simulink model "estimator"  (R2024a)
settings: Solver=FixedStepAuto  StartTime=0.0  StopTime=400  FixedStep=0.001  RelTol=1e-3
InitFcn:
  | Kx = 20;
  | Kf = 21;
settings Model: Creator=bemran  LastModifiedBy=bemran

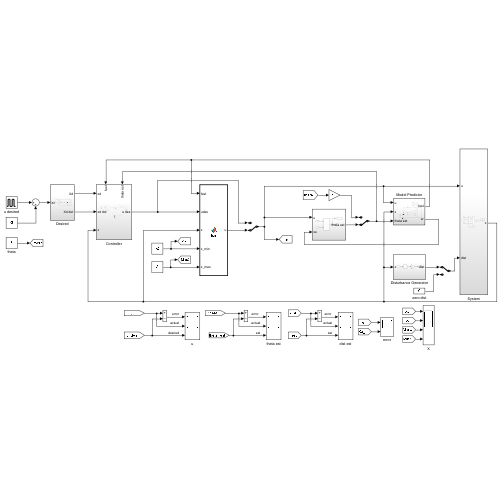
[thumbnail: Simulink's stored preview of the top-level diagram]
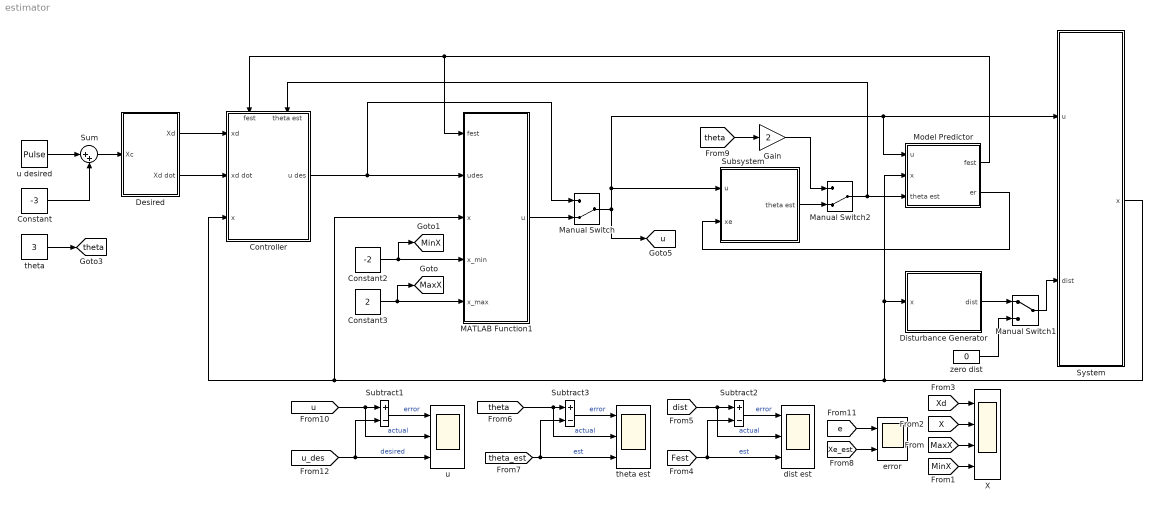
== system estimator ==
  Constant : Constant  Value=-3
  Constant2 : Constant  Value=-2
  Constant3 : Constant  Value=2
  Controller : Subsystem
      settings: PortSchema="{\"entries\":[{\"content\":{\"sides\":[{\"content\":{\"connectorIds\":[\"In1\",\"In2\",\"In3\"]},\"type\":\"ConnectorPlacement.EquallySpacedRectSide\",\"uuid\":\"b6f38cdc-8bf3-4480-b58d-f3be2425ec5d\"},{\"content\":{\"connectorIds\":[\"Out1\"],\"side\":\"RIGHT\"},\"type\":\"ConnectorPlacement.EquallySpacedRectSide\",\"uuid\":\"bcaedb91-bba6-4987-806b-aba45422edc9\"},{\"content\":{\"connectorIds\":[\"In4\",\"In5\"],\"side\":\"TOP\"},\"type\":\"ConnectorPlacement.EquallySpacedRectSide\",\"uuid\":\"b280daf0-8ac8-4898-b226-e1ec0883028d\"},{\"content\":{\"side\":\"BOTTOM\"},\"type\":\"ConnectorPlacement.EquallySpacedRectSide\",\"uuid\":\"a3314033-a6b2-4450-a5a3-9d51c6c5191b\"}]},\"type\":\"ConnectorPlacement.EquallySpacedConnector\",\"uuid\":\"d4e8f3f5-abab-496a-b317-e8d184215eb1\"}],\"packageUris\":[\"http://schema.mathworks.com/mf0/Connector/R2020b\"],\"version\":\"1.0\"}"
  Desired : Subsystem
  Disturbance Generator : Subsystem
  Gain : Gain  Gain=2
  MATLAB Function1 : MATLAB Function  TreatAsAtomicUnit=on
  Manual Switch : ManualSwitch  CurrentSetting=0
  Manual Switch1 : ManualSwitch
  Manual Switch2 : ManualSwitch  CurrentSetting=0
  Model Predictor : Subsystem
      settings: PortSchema="{\"entries\":[{\"content\":{\"sides\":[{\"content\":{\"connectorIds\":[\"Out1\",\"Out2\"]},\"type\":\"ConnectorPlacement.EquallySpacedRectSide\",\"uuid\":\"6e6569c2-bc7f-4167-ae98-e66125c9e1e3\"},{\"content\":{\"connectorIds\":[\"In1\",\"In2\",\"In3\"],\"side\":\"RIGHT\"},\"type\":\"ConnectorPlacement.EquallySpacedRectSide\",\"uuid\":\"af0deaad-808c-4137-9b9d-c847525b3dac\"},{\"content\":{\"side\":\"TOP\"},\"type\":\"ConnectorPlacement.EquallySpacedRectSide\",\"uuid\":\"ed017cdd-fa89-4299-a174-caff2025e69e\"}]},\"type\":\"ConnectorPlacement.EquallySpacedConnector\",\"uuid\":\"feb2a9a1-0b16-4155-b32e-177a30695464\"}],\"packageUris\":[\"http://schema.mathworks.com/mf0/Connector/R2020b\"],\"version\":\"1.0\"}"
  Subsystem : Subsystem
  Subtract1 : Sum  Inputs=+-
  Subtract2 : Sum  Inputs=+-
  Subtract3 : Sum  Inputs=+-
  Sum : Sum  Inputs=|++
  System : Subsystem
  X : Scope  NumInputPorts=4
  dist est : Scope  NumInputPorts=3
  error : Scope  NumInputPorts=2
  theta : Constant  Value=3
  theta est : Scope  NumInputPorts=3
  u : Scope  NumInputPorts=3
  u desired : DiscretePulseGenerator  PulseType=Time based  Amplitude=6  Period=40  PulseWidth=50
  zero dist : Constant  Value=0
  tag scope: MaxX=global, MinX=global, theta=global, u=global
  wires:
  u desired/1 -> Sum/1
  Constant/1 -> Sum/2
  Sum/1 -> Desired/1(Xc)
  Constant3/1 -> [MaxX], MATLAB Function1/5(x_max)
  Constant2/1 -> MATLAB Function1/4(x_min), [MinX]
  [MaxX] -> X/3
  [MinX] -> X/4
  [X] -> X/2
  [Xd] -> X/1
  Manual Switch1/1 -> System/2(dist)
  Disturbance Generator/1(dist) -> Manual Switch1/1
  zero dist/1 -> Manual Switch1/2
  System/1(x) -> MATLAB Function1/3(x), Controller/3(x), Model Predictor/2(x), Disturbance Generator/1(x)
  Manual Switch/1 -> [u], Model Predictor/1(u), System/1(u), Subsystem/1(u)
  Model Predictor/1(fest) -> Controller/4(fest), MATLAB Function1/1(fest)
  Subtract3/1 -> theta est/1  "error"
  [theta] -> theta est/2, Subtract3/1  "actual"
  [theta_est] -> theta est/3, Subtract3/2  "est"
  MATLAB Function1/1(u) -> Manual Switch/2
  Controller/1(u des) -> MATLAB Function1/2(udes), Manual Switch/1
  [e] -> error/1
  theta/1 -> [theta]
  [Fest] -> dist est/3, Subtract2/2  "est"
  Subtract2/1 -> dist est/1  "error"
  [dist] -> dist est/2, Subtract2/1  "actual"
  [u_des] -> u/3, Subtract1/2  "desired"
  [u] -> u/2, Subtract1/1  "actual"
  Subtract1/1 -> u/1  "error"
  Desired/1(Xd) -> Controller/1(xd)
  Desired/2(Xd dot) -> Controller/2(xd dot)
  Manual Switch2/1 -> Model Predictor/3(theta est), Controller/5(theta est)
  Model Predictor/2(er) -> Subsystem/2(xe)
  [Xe_est] -> error/2
  [theta] -> Gain/1
  Subsystem/1(theta est) -> Manual Switch2/2
  Gain/1 -> Manual Switch2/1

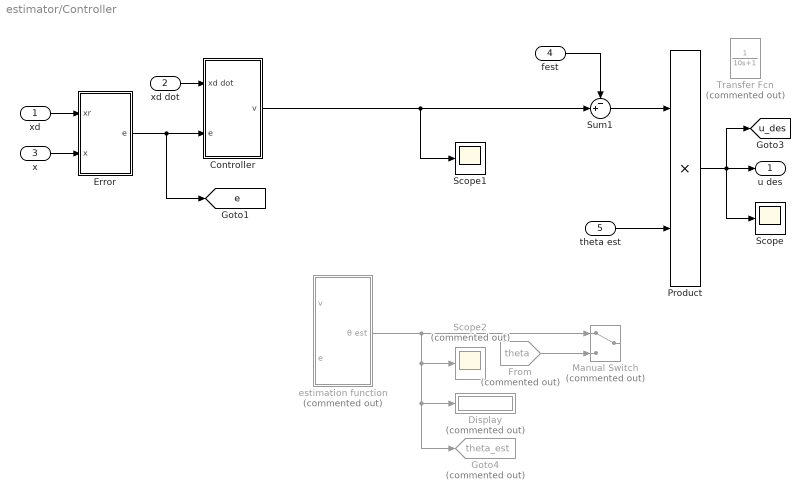
== system estimator/Controller ==
  xd : Inport
  xd dot : Inport  Port=2
  x : Inport  Port=3
  fest : Inport  Port=4
  theta est : Inport  Port=5
  Controller : Subsystem
  Display : Display  Commented=on
  Error : Subsystem
  From : From  Commented=on  GotoTag=theta  TagVisibility=global
  Goto4 : Goto  Commented=on  GotoTag=theta_est  TagVisibility=global
  Manual Switch : ManualSwitch  Commented=on
  Product : Product  Inputs=**
  Scope : Scope
  Scope1 : Scope
  Scope2 : Scope  Commented=on
  Sum1 : Sum  Inputs=-+|
  Transfer Fcn : TransferFcn  Commented=on  Denominator=[10 1]
  estimation function : Subsystem  Commented=on  mask{gamma=0.1, MaxEstiamtedTheta=4, MinEstiamtedTheta=0.1, InertiaInitialCondition=1.2}
      mask prompts: MaxEstiamtedTheta "Maximum Estiamted Theta"; MinEstiamtedTheta "Minimum Estiamted Theta"; InertiaInitialCondition "Inertia Initial Condition"
      mask TypeOptions gamma: gama/Gain
      mask TypeOptions MaxEstiamtedTheta: θ Max/Value
      mask TypeOptions MinEstiamtedTheta: θ Min/Value
      mask TypeOptions InertiaInitialCondition: θ estimate/InitialCondition
      mask DialogControl Container Prompt: Estimation Paraemter
  u des : Outport
  tag scope: e=global, u_des=global
  wires:
  fest/1 -> Sum1/1
  Sum1/1 -> Product/1
  estimation function/1("  θ est") -> Goto4/1, Display/1, Scope2/1, Manual Switch/1
  xd/1 -> Error/1(xr)
  x/1 -> Error/2(x)
  Product/1 -> [u_des], Scope/1, u des/1
  theta est/1 -> Product/2
  From/1 -> Manual Switch/2
  xd dot/1 -> Controller/1(xd dot)
  Error/1(e) -> [e], Controller/2(e)
  Controller/1(v) -> Scope1/1, Sum1/2

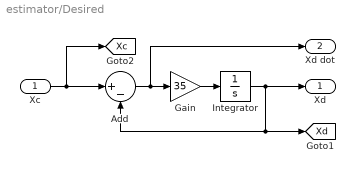
== system estimator/Desired ==
  Xc : Inport
  Add : Sum  Inputs=|+-
  Gain : Gain  Gain=35
  Integrator : Integrator
  Xd : Outport
  Xd dot : Outport  Port=2
  tag scope: Xc=global, Xd=global
  wires:
  Gain/1 -> Integrator/1
  Integrator/1 -> Xd/1, [Xd], Add/2
  Add/1 -> Xd dot/1, Gain/1
  Xc/1 -> [Xc], Add/1

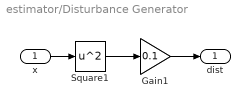
== system estimator/Disturbance Generator ==
  x : Inport
  Gain1 : Gain  Gain=0.1
  Square1 : Math  Operator=square
  dist : Outport
  wires:
  Gain1/1 -> dist/1
  Square1/1 -> Gain1/1
  x/1 -> Square1/1

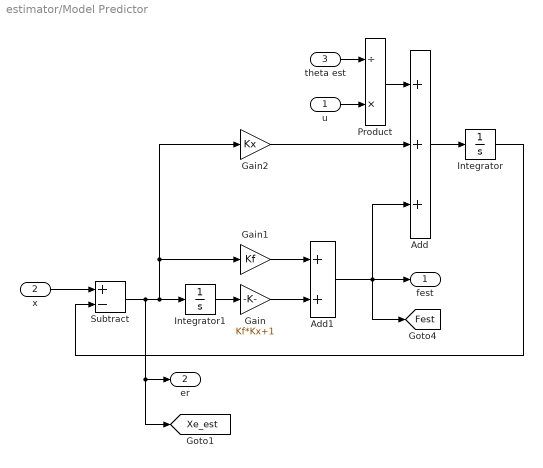
== system estimator/Model Predictor ==
  u : Inport
  x : Inport  Port=2
  theta est : Inport  Port=3
  Add : Sum  Inputs=+++
  Add1 : Sum
  Gain : Gain  Gain=Kf*Kx+1
  Gain1 : Gain  Gain=Kf
  Gain2 : Gain  Gain=Kx
  Integrator : Integrator
  Integrator1 : Integrator
  Product : Product  Inputs=/*
  Subtract : Sum  Inputs=+-
  fest : Outport
  er : Outport  Port=2
  tag scope: Fest=global, Xe_est=global
  wires:
  Add/1 -> Integrator/1
  x/1 -> Subtract/1
  Integrator1/1 -> Gain/1
  Gain/1 -> Add1/2
  Gain1/1 -> Add1/1
  Gain2/1 -> Add/2
  Integrator/1 -> Subtract/2
  Add1/1 -> [Fest], fest/1, Add/3
  Subtract/1 -> er/1, [Xe_est], Gain1/1, Gain2/1, Integrator1/1
  Product/1 -> Add/1
  theta est/1 -> Product/1
  u/1 -> Product/2

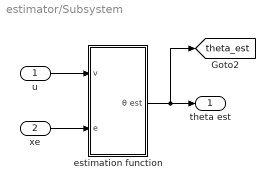
== system estimator/Subsystem ==
  u : Inport
  xe : Inport  Port=2
  estimation function : Subsystem  mask{gamma=1, MaxEstiamtedTheta=4, MinEstiamtedTheta=0.1, InertiaInitialCondition=1.2}
      mask prompts: MaxEstiamtedTheta "Maximum Estiamted Theta"; MinEstiamtedTheta "Minimum Estiamted Theta"; InertiaInitialCondition "Inertia Initial Condition"
      mask TypeOptions gamma: gama/Gain
      mask TypeOptions MaxEstiamtedTheta: θ Max/Value
      mask TypeOptions MinEstiamtedTheta: θ Min/Value
      mask TypeOptions InertiaInitialCondition: θ estimate/InitialCondition
      mask DialogControl Container Prompt: Estimation Paraemter
  theta est : Outport
  tag scope: theta_est=global
  wires:
  u/1 -> estimation function/1(v)
  estimation function/1("  θ est") -> theta est/1, [theta_est]
  xe/1 -> estimation function/2(e)

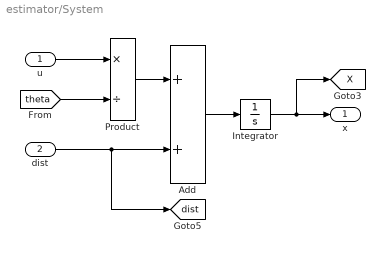
== system estimator/System ==
  u : Inport
  dist : Inport  Port=2
  Add : Sum
  Integrator : Integrator
  Product : Product  Inputs=*/
  x : Outport
  tag scope: X=global, dist=global
  wires:
  u/1 -> Product/1
  Add/1 -> Integrator/1
  dist/1 -> [dist], Add/2
  Product/1 -> Add/1
  Integrator/1 -> [X], x/1
  [theta] -> Product/2

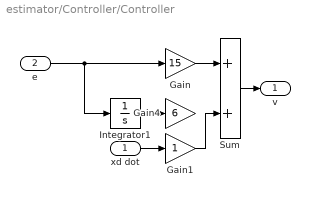
== system estimator/Controller/Controller ==
  xd dot : Inport
  e : Inport  Port=2
  Gain : Gain  Gain=15
  Gain1 : Gain
  Gain4 : Gain  Gain=6
  Integrator1 : Integrator  InitialCondition=1
  Sum : Sum
  v : Outport
  wires:
  Sum/1 -> v/1
  Gain/1 -> Sum/1
  Integrator1/1 -> Gain4/1
  e/1 -> Integrator1/1, Gain/1
  xd dot/1 -> Gain1/1
  Gain1/1 -> Sum/2

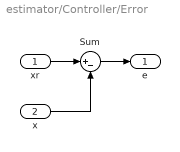
== system estimator/Controller/Error ==
  xr : Inport
  x : Inport  Port=2
  Sum : Sum  Inputs=|+-
  e : Outport
  wires:
  x/1 -> Sum/2
  xr/1 -> Sum/1
  Sum/1 -> e/1

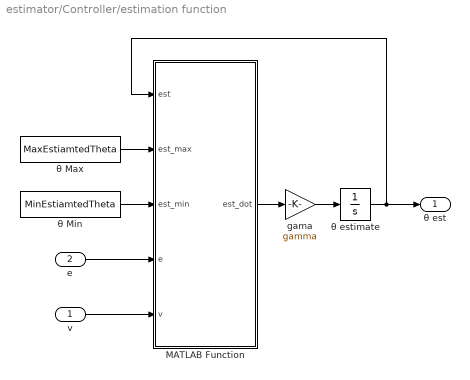
== system estimator/Controller/estimation function ==
  v : Inport
  e : Inport  Port=2
  MATLAB Function : MATLAB Function  TreatAsAtomicUnit=on
  gama : Gain  Gain=gamma
  θ Max : Constant  Value=MaxEstiamtedTheta
  θ Min : Constant  Value=MinEstiamtedTheta
  θ estimate : Integrator  InitialCondition=InertiaInitialCondition  LimitOutput=on  UpperSaturationLimit=MaxEstiamtedTheta  LowerSaturationLimit=MinEstiamtedTheta
  "  θ est" : Outport
  wires:
  gama/1 -> θ estimate/1
  θ Max/1 -> MATLAB Function/2(est_max)
  θ Min/1 -> MATLAB Function/3(est_min)
  θ estimate/1 -> MATLAB Function/1(est), "  θ est"/1
  MATLAB Function/1(est_dot) -> gama/1
  v/1 -> MATLAB Function/5(v)
  e/1 -> MATLAB Function/4(e)

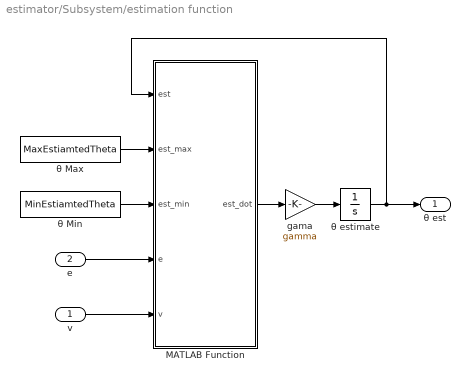
== system estimator/Subsystem/estimation function ==
  v : Inport
  e : Inport  Port=2
  MATLAB Function : MATLAB Function  TreatAsAtomicUnit=on
  gama : Gain  Gain=gamma
  θ Max : Constant  Value=MaxEstiamtedTheta
  θ Min : Constant  Value=MinEstiamtedTheta
  θ estimate : Integrator  InitialCondition=InertiaInitialCondition  LimitOutput=on  UpperSaturationLimit=MaxEstiamtedTheta  LowerSaturationLimit=MinEstiamtedTheta
  "  θ est" : Outport
  wires:
  gama/1 -> θ estimate/1
  θ Max/1 -> MATLAB Function/2(est_max)
  θ Min/1 -> MATLAB Function/3(est_min)
  θ estimate/1 -> MATLAB Function/1(est), "  θ est"/1
  MATLAB Function/1(est_dot) -> gama/1
  v/1 -> MATLAB Function/5(v)
  e/1 -> MATLAB Function/4(e)

== matlab function estimator/MATLAB Function1 ==
  data: fest input; udes input; u output; x input; x_min input; x_max input
function u = fcn(fest, udes, x, x_min, x_max)
% h1 = (xmax - x) >= 0 
%h1dot = -xdot >= - alpha (xmax - x) => u <= alpha (xmax - x)
% h2 = (x- xmin) >= 0 
%h2dot = xdot >= - alpha (x - xmin) => - u <= alpha (x - xmin)
% J = (u-udes)^2 -> J = u^2 - 2*udes*u + udes^2 
% J = 1/2 x' * H * x + f' x;
% A*x <= b
%We have two conditions:
%   u <= alpha (xmax-x)
% -u <= alpha (x - xmin)

H = [2]; 
f = [-2 * udes];
A = [1;
     -1];
alpha = 10; 
F = fest;%0.5 * x^2;
b = [- F + alpha*(x_max-x); 
      + F + alpha*(x-x_min)];
options = optimoptions('quadprog','Algorithm','active-set');
[u_opt] =  quadprog(H, f, A, b, [], [], [], [], udes, options);
% if(exitflag == 1)
    u = u_opt;
% else
    % u = 0;
% end

== matlab function estimator/Subsystem/estimation function/MATLAB Function ==
  data: est_dot output size=[1]; est input size=[1]; est_max input size=[1]; est_min input size=[1]; e input size=[1]; v input size=[1]
function est_dot = fcn(est, est_max, est_min, e, v)
est_dot_tmp = - v * e';
est_dot = zeros(size(est));

if norm(e) > 0.01
    for i = 1:length(est(:))
        est_dot(i) = EstDot(est_dot_tmp(i), est(i), est_max(i), est_min(i));
    end
end

function est_dot = EstDot(tmp, est, est_max, est_min)
  est_dot = 0;
  if (est < est_max && est > est_min) || ...
      (est > est_min && tmp < 0) || ...
      (est < est_max && tmp > 0) 
        est_dot = tmp;
  end 
end

end

== matlab function estimator/Controller/estimation function/MATLAB Function ==
  data: est_dot output size=[1]; est input size=[1]; est_max input size=[1]; est_min input size=[1]; e input size=[1]; v input size=[1]
function est_dot = fcn(est, est_max, est_min, e, v)
est_dot_tmp = - v * e';
est_dot = zeros(size(est));

if norm(e) > 0.01
    for i = 1:length(est(:))
        est_dot(i) = EstDot(est_dot_tmp(i), est(i), est_max(i), est_min(i));
    end
end

function est_dot = EstDot(tmp, est, est_max, est_min)
  est_dot = 0;
  if (est < est_max && est > est_min) || ...
      (est > est_min && tmp < 0) || ...
      (est < est_max && tmp > 0) 
        est_dot = tmp;
  end 
end

end
